simulink library "VentilatorLibrary"  (R2019b)
settings: Solver=VariableStepAuto  StartTime=0.0  StopTime=10.0  RelTol=1e-3
PreLoadFcn:
  | % Conversion factors
  | cmH2O_to_Pa = 98.0665;
  | L_to_m3 = 1e-3;
  | 
  | % Load thermodynamic data of N2, O2 and water vapor
  | load moistAirProperties
undefined symbols (not defined in the file): D_tube
libraries: fl_lib x109, simulink x2, HVAC_lib x1, nesl_utility x1
(part 2 of 2)

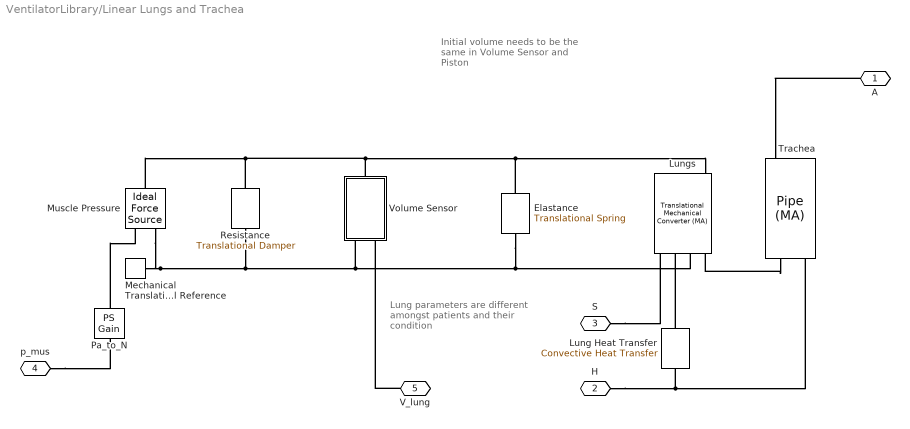
== system VentilatorLibrary/Linear Lungs and Trachea ==
  note: Lung parameters
      | are different
      | amongst patients
      | and their condition
  note: Initial volume needs
      | to be the same in
      | Volume Sensor
      | and Piston
  Elastance : fl_lib/Mechanical/Translational Elements/Translational Spring  spr_rate=E_respiratory*cmH2O_to_Pa/L_to_m3*A_interface^2 N/m  v_specify=off  v_priority=None  v=0 m/s  v_nominal_specify=off  v_nominal_unit=m/s  v_nominal_value=1  f_specify=off  f_priority=None  f=0 N  f_nominal_specify=off  f_nominal_unit=N  f_nominal_value=1  x_specify=on  x_priority=High  x=(vol_init - FRC)*L_to_m3/A_interface m  x_nominal_specify=off  x_nominal_unit=m  x_nominal_value=1
  Lung Heat Transfer : fl_lib/Thermal/Thermal Elements/Convective Heat Transfer  area=80 m^2  heat_tr_coeff=20 W/(m^2 * K)  T_specify=off  T_priority=None  T=0 K  T_nominal_specify=off  T_nominal_unit=K  T_nominal_value=1  Q_specify=off  Q_priority=None  Q=0 W  Q_nominal_specify=off  Q_nominal_unit=W  Q_nominal_value=1
  Lungs : fl_lib/Moist Air/Elements/Translational Mechanical Converter (MA)  mech_orientation=simscape.enum.posneg.positive  interface_area=A_interface m^2  length_init=vol_init* L_to_m3/A_interface m  dead_volume=1e-6 m^3  area_A=pi*D_trachea^2/4 m^2  pressure_spec=foundation.enum.pressure_spec.atmospheric  environment_pressure=0.101325 MPa  RH_ws=1  time_constant=1e-3 s  moisture_trace_gas_source=foundation.enum.moisture_trace_gas_source.controlled  moisture_source_spec=foundation.enum.moisture_source_spec.vapor  moisture_mass_flow=0 kg/s  moisture_temperature_spec=foundation.enum.temperature_spec.atmospheric  moisture_temperature=293.15 K  trace_gas_mass_flow=0 kg/s  trace_gas_temperature_spec=foundation.enum.temperature_spec.atmospheric  trace_gas_temperature=293.15 K  p_I_specify=on  p_I_priority=None  p_I=0.101325 MPa  p_I_nominal_specify=off  p_I_nominal_unit=MPa  p_I_nominal_value=1  T_I_specify=on  T_I_priority=High  T_I=T_init degC  T_I_nominal_specify=off  T_I_nominal_unit=K  T_I_nominal_value=1  RH_I_specify=on  RH_I_priority=High  RH_I=1  RH_I_nominal_specify=off  RH_I_nominal_unit=1  RH_I_nominal_value=1  x_w_I_specify=off  x_w_I_priority=None  x_w_I=0  x_w_I_nominal_specify=off  x_w_I_nominal_unit=1  x_w_I_nominal_value=1  y_w_I_specify=off  y_w_I_priority=None  y_w_I=0  y_w_I_nominal_specify=off  y_w_I_nominal_unit=1  y_w_I_nominal_value=1  HR_I_specify=off  HR_I_priority=None  HR_I=0  HR_I_nominal_specify=off  HR_I_nominal_unit=1  HR_I_nominal_value=1  x_g_I_specify=on  x_g_I_priority=None  x_g_I=0  x_g_I_nominal_specify=off  x_g_I_nominal_unit=1  x_g_I_nominal_value=1  y_g_I_specify=on  y_g_I_priority=High  y_g_I=0.7  y_g_I_nominal_specify=off  y_g_I_nominal_unit=1  y_g_I_nominal_value=1
      settings: SourceProductName=Simscape  SourceProductBaseCode=SS  InternalSimscapePortConfiguration="{\"Bottom\":[],\"Left\":[{\"id\":\"A\",\"label\":\"A\",\"type\":\"foundation.moist_air.moist_air\"},{\"id\":\"C\",\"label\":\"C\",\"type\":\"foundation.mechanical.translational.translational\"},{\"id\":\"H\",\"label\":\"H\",\"type\":\"foundation.thermal.thermal\"},{\"id\":\"S\",\"label\":\"S\",\"type\":\"foundation.moist_air.moist_air_source\"}],\"Right\":[{\"id\":\"R\",\"label\":\"R\",\"type\":\"foundation.mechanical.translational.translational\"},{\"id\":\"W\",\"label\":\"W\",\"type\":\"output\"},{\"id\":\"F\",\"label\":\"F\",\"type\":\"output\"}],\"Top\":[]}"
  Mechanical Translational Reference : fl_lib/Mechanical/Translational Elements/Mechanical Translational Reference
  Muscle Pressure : fl_lib/Mechanical/Mechanical Sources/Ideal Force Source
  Pa_to_N : fl_lib/Physical Signals/Functions/PS Gain  gain=A_interface N/Pa
  Resistance : fl_lib/Mechanical/Translational Elements/Translational Damper  D=(R_respiratory * cmH2O_to_Pa/ L_to_m3)*A_interface^2 N/(m/s)  v_specify=off  v_priority=None  v=0 m/s  v_nominal_specify=off  v_nominal_unit=m/s  v_nominal_value=1  f_specify=off  f_priority=None  f=0 N  f_nominal_specify=off  f_nominal_unit=N  f_nominal_value=1
  Trachea : fl_lib/Moist Air/Elements/Pipe (MA)  length=L_trachea m  area=pi*D_trachea^2/4 m^2  Dh=D_trachea m  length_add=0.1 m  roughness=15e-6 m  Re_lam=2000  Re_tur=4000  shape_factor=64  Nu_lam=3.66  RH_ws=1  time_constant=1e-3 s  moisture_trace_gas_source=foundation.enum.moisture_trace_gas_source.none  moisture_source_spec=foundation.enum.moisture_source_spec.vapor  moisture_mass_flow=0 kg/s  moisture_temperature_spec=foundation.enum.temperature_spec.atmospheric  moisture_temperature=293.15 K  trace_gas_mass_flow=0 kg/s  trace_gas_temperature_spec=foundation.enum.temperature_spec.atmospheric  trace_gas_temperature=293.15 K  p_I_specify=on  p_I_priority=None  p_I=0.101325 MPa  p_I_nominal_specify=off  p_I_nominal_unit=MPa  p_I_nominal_value=1  T_I_specify=on  T_I_priority=High  T_I=T_init degC  T_I_nominal_specify=off  T_I_nominal_unit=K  T_I_nominal_value=1  RH_I_specify=on  RH_I_priority=High  RH_I=1  RH_I_nominal_specify=off  RH_I_nominal_unit=1  RH_I_nominal_value=1  x_w_I_specify=off  x_w_I_priority=None  x_w_I=0  x_w_I_nominal_specify=off  x_w_I_nominal_unit=1  x_w_I_nominal_value=1  y_w_I_specify=off  y_w_I_priority=None  y_w_I=0  y_w_I_nominal_specify=off  y_w_I_nominal_unit=1  y_w_I_nominal_value=1  HR_I_specify=off  HR_I_priority=None  HR_I=0  HR_I_nominal_specify=off  HR_I_nominal_unit=1  HR_I_nominal_value=1  x_g_I_specify=on  x_g_I_priority=None  x_g_I=0  x_g_I_nominal_specify=off  x_g_I_nominal_unit=1  x_g_I_nominal_value=1  y_g_I_specify=on  y_g_I_priority=High  y_g_I=0.7  y_g_I_nominal_specify=off  y_g_I_nominal_unit=1  y_g_I_nominal_value=1
      settings: SourceProductName=Simscape  SourceProductBaseCode=SS
  Volume Sensor : Subsystem  mask(Volume Data){vol_init=vol_init}
      mask prompts: vol_init "Initial lung volume [L]"
      mask help: This subsystem reports the lung volume. Because the Interface cross-sectional area parameter in the lung model is set to 1 m^2, therefore 1 m of measured displacement is equivalent to 1 m^3 of lung volume and 1 N of measured force is equivalent to 1 Pa of pressure.
      mask init:
      | L_to_m3 = 1e-3;
  A : PMIOPort  Side=Right
  H : PMIOPort  Port=2  Side=Left
  S : PMIOPort  Port=3  Side=Left
  p_mus : PMIOPort  Port=4  Side=Left
  V_lung : PMIOPort  Port=5  Side=Right
  connections:
  Pa_to_N/RConn1 -- Muscle Pressure/RConn1
  p_mus/RConn1 -- Pa_to_N/LConn1
  V_lung/RConn1 -- Volume Sensor/RConn2
  S/RConn1 -- Lungs/LConn4
  A/RConn1 -- Trachea/RConn1
  Volume Sensor/RConn1 -- Resistance/RConn1 -- Muscle Pressure/RConn2 -- Mechanical Translational Reference/LConn1 -- Elastance/RConn1 -- Lungs/LConn2
  Lung Heat Transfer/LConn1 -- Lungs/LConn3
  Trachea/LConn2 -- Lung Heat Transfer/RConn1 -- H/RConn1
  Resistance/LConn1 -- Muscle Pressure/LConn1 -- Volume Sensor/LConn1 -- Elastance/LConn1 -- Lungs/RConn1
  Trachea/LConn1 -- Lungs/LConn1

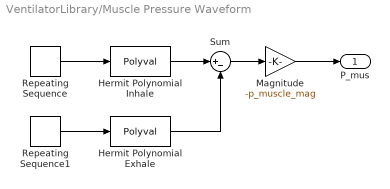
== system VentilatorLibrary/Muscle Pressure Waveform ==
  Hermit Polynomial Exhale : Polyval  Coefs=[-2, 3, 0, 0]
  Hermit Polynomial Inhale : Polyval  Coefs=[-2, 3, 0, 0]
  Magnitude : Gain  Gain=-p_muscle_mag
  Repeating Sequence : simulink/Sources/Repeating Sequence  rep_seq_t=[0, t_inhale, period]  rep_seq_y=[0, 1, 1]
  Repeating Sequence1 : simulink/Sources/Repeating Sequence  rep_seq_t=[0, t_inhale, t_inhale+t_exhale, period]  rep_seq_y=[0, 0, 1, 1]
  Sum : Sum  Inputs=|+-
  P_mus : Outport  VectorParamsAs1DForOutWhenUnconnected=off
  wires:
  Magnitude/1 -> P_mus/1
  Hermit Polynomial Inhale/1 -> Sum/1
  Repeating Sequence/1 -> Hermit Polynomial Inhale/1
  Repeating Sequence1/1 -> Hermit Polynomial Exhale/1
  Sum/1 -> Magnitude/1
  Hermit Polynomial Exhale/1 -> Sum/2

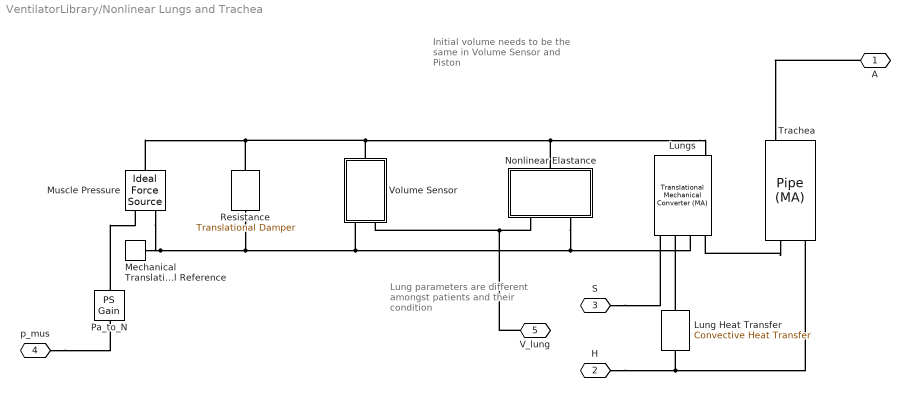
== system VentilatorLibrary/Nonlinear Lungs and Trachea ==
  note: Initial volume needs
      | to be the same in
      | Volume Sensor
      | and Piston
  note: Lung parameters
      | are different
      | amongst patients
      | and their condition
  Lung Heat Transfer : fl_lib/Thermal/Thermal Elements/Convective Heat Transfer  area=80 m^2  heat_tr_coeff=20 W/(m^2 * K)  T_specify=off  T_priority=None  T=0 K  T_nominal_specify=off  T_nominal_unit=K  T_nominal_value=1  Q_specify=off  Q_priority=None  Q=0 W  Q_nominal_specify=off  Q_nominal_unit=W  Q_nominal_value=1
  Lungs : fl_lib/Moist Air/Elements/Translational Mechanical Converter (MA)  mech_orientation=simscape.enum.posneg.positive  interface_area=A_interface m^2  length_init=vol_init* L_to_m3/A_interface m  dead_volume=1e-6 m^3  area_A=pi*D_trachea^2/4 m^2  pressure_spec=foundation.enum.pressure_spec.atmospheric  environment_pressure=0.101325 MPa  RH_ws=1  time_constant=1e-3 s  moisture_trace_gas_source=foundation.enum.moisture_trace_gas_source.controlled  moisture_source_spec=foundation.enum.moisture_source_spec.vapor  moisture_mass_flow=0 kg/s  moisture_temperature_spec=foundation.enum.temperature_spec.atmospheric  moisture_temperature=293.15 K  trace_gas_mass_flow=0 kg/s  trace_gas_temperature_spec=foundation.enum.temperature_spec.atmospheric  trace_gas_temperature=293.15 K  p_I_specify=on  p_I_priority=None  p_I=0.101325 MPa  p_I_nominal_specify=off  p_I_nominal_unit=MPa  p_I_nominal_value=1  T_I_specify=on  T_I_priority=High  T_I=T_init degC  T_I_nominal_specify=off  T_I_nominal_unit=K  T_I_nominal_value=1  RH_I_specify=on  RH_I_priority=High  RH_I=1  RH_I_nominal_specify=off  RH_I_nominal_unit=1  RH_I_nominal_value=1  x_w_I_specify=off  x_w_I_priority=None  x_w_I=0  x_w_I_nominal_specify=off  x_w_I_nominal_unit=1  x_w_I_nominal_value=1  y_w_I_specify=off  y_w_I_priority=None  y_w_I=0  y_w_I_nominal_specify=off  y_w_I_nominal_unit=1  y_w_I_nominal_value=1  HR_I_specify=off  HR_I_priority=None  HR_I=0  HR_I_nominal_specify=off  HR_I_nominal_unit=1  HR_I_nominal_value=1  x_g_I_specify=on  x_g_I_priority=None  x_g_I=0  x_g_I_nominal_specify=off  x_g_I_nominal_unit=1  x_g_I_nominal_value=1  y_g_I_specify=on  y_g_I_priority=High  y_g_I=0.7  y_g_I_nominal_specify=off  y_g_I_nominal_unit=1  y_g_I_nominal_value=1
      settings: SourceProductName=Simscape  SourceProductBaseCode=SS  InternalSimscapePortConfiguration="{\"Bottom\":[],\"Left\":[{\"id\":\"A\",\"label\":\"A\",\"type\":\"foundation.moist_air.moist_air\"},{\"id\":\"C\",\"label\":\"C\",\"type\":\"foundation.mechanical.translational.translational\"},{\"id\":\"H\",\"label\":\"H\",\"type\":\"foundation.thermal.thermal\"},{\"id\":\"S\",\"label\":\"S\",\"type\":\"foundation.moist_air.moist_air_source\"}],\"Right\":[{\"id\":\"R\",\"label\":\"R\",\"type\":\"foundation.mechanical.translational.translational\"},{\"id\":\"W\",\"label\":\"W\",\"type\":\"output\"},{\"id\":\"F\",\"label\":\"F\",\"type\":\"output\"}],\"Top\":[]}"
  Mechanical Translational Reference : fl_lib/Mechanical/Translational Elements/Mechanical Translational Reference
  Muscle Pressure : fl_lib/Mechanical/Mechanical Sources/Ideal Force Source
  Nonlinear Elastance : Subsystem  mask{Vmax=Vmax, E_respiratory=E_respiratory, FRC=FRC}
      mask prompts: Vmax "Lung capacity [L]:"; E_respiratory "Elastance at equilibrium volume [cmH2O/L]"; FRC "Functional Residual Capacity (equilibrium volume) [L]:"
      mask Display: disp('F=k2*tan(k1*x)')
  Pa_to_N : fl_lib/Physical Signals/Functions/PS Gain  gain=A_interface N/Pa
  Resistance : fl_lib/Mechanical/Translational Elements/Translational Damper  D=(R_respiratory * cmH2O_to_Pa/ L_to_m3)*A_interface^2 N/(m/s)  v_specify=off  v_priority=None  v=0 m/s  v_nominal_specify=off  v_nominal_unit=m/s  v_nominal_value=1  f_specify=off  f_priority=None  f=0 N  f_nominal_specify=off  f_nominal_unit=N  f_nominal_value=1
  Trachea : fl_lib/Moist Air/Elements/Pipe (MA)  length=L_trachea m  area=pi*D_trachea^2/4 m^2  Dh=D_trachea m  length_add=0.1 m  roughness=15e-6 m  Re_lam=2000  Re_tur=4000  shape_factor=64  Nu_lam=3.66  RH_ws=1  time_constant=1e-3 s  moisture_trace_gas_source=foundation.enum.moisture_trace_gas_source.none  moisture_source_spec=foundation.enum.moisture_source_spec.vapor  moisture_mass_flow=0 kg/s  moisture_temperature_spec=foundation.enum.temperature_spec.atmospheric  moisture_temperature=293.15 K  trace_gas_mass_flow=0 kg/s  trace_gas_temperature_spec=foundation.enum.temperature_spec.atmospheric  trace_gas_temperature=293.15 K  p_I_specify=on  p_I_priority=None  p_I=0.101325 MPa  p_I_nominal_specify=off  p_I_nominal_unit=MPa  p_I_nominal_value=1  T_I_specify=on  T_I_priority=High  T_I=T_init degC  T_I_nominal_specify=off  T_I_nominal_unit=K  T_I_nominal_value=1  RH_I_specify=on  RH_I_priority=High  RH_I=1  RH_I_nominal_specify=off  RH_I_nominal_unit=1  RH_I_nominal_value=1  x_w_I_specify=off  x_w_I_priority=None  x_w_I=0  x_w_I_nominal_specify=off  x_w_I_nominal_unit=1  x_w_I_nominal_value=1  y_w_I_specify=off  y_w_I_priority=None  y_w_I=0  y_w_I_nominal_specify=off  y_w_I_nominal_unit=1  y_w_I_nominal_value=1  HR_I_specify=off  HR_I_priority=None  HR_I=0  HR_I_nominal_specify=off  HR_I_nominal_unit=1  HR_I_nominal_value=1  x_g_I_specify=on  x_g_I_priority=None  x_g_I=0  x_g_I_nominal_specify=off  x_g_I_nominal_unit=1  x_g_I_nominal_value=1  y_g_I_specify=on  y_g_I_priority=High  y_g_I=0.7  y_g_I_nominal_specify=off  y_g_I_nominal_unit=1  y_g_I_nominal_value=1
      settings: SourceProductName=Simscape  SourceProductBaseCode=SS
  Volume Sensor : Subsystem  mask(Volume Data){vol_init=vol_init}
      mask prompts: vol_init "Initial lung volume [L]"
      mask help: This subsystem reports the lung volume. Because the Interface cross-sectional area parameter in the lung model is set to 1 m^2, therefore 1 m of measured displacement is equivalent to 1 m^3 of lung volume and 1 N of measured force is equivalent to 1 Pa of pressure.
      mask init:
      | L_to_m3 = 1e-3
  A : PMIOPort  Side=Right
  H : PMIOPort  Port=2  Side=Left
  S : PMIOPort  Port=3  Side=Left
  p_mus : PMIOPort  Port=4  Side=Left
  V_lung : PMIOPort  Port=5  Side=Right
  connections:
  Trachea/LConn1 -- Lungs/LConn1
  Lungs/RConn1 -- Volume Sensor/LConn1 -- Muscle Pressure/LConn1 -- Resistance/LConn1 -- Nonlinear Elastance/LConn1
  H/RConn1 -- Lung Heat Transfer/RConn1 -- Trachea/LConn2
  Lung Heat Transfer/LConn1 -- Lungs/LConn3
  Lungs/LConn2 -- Mechanical Translational Reference/LConn1 -- Muscle Pressure/RConn2 -- Resistance/RConn1 -- Volume Sensor/RConn1 -- Nonlinear Elastance/RConn2
  A/RConn1 -- Trachea/RConn1
  S/RConn1 -- Lungs/LConn4
  Nonlinear Elastance/RConn1 -- Volume Sensor/RConn2 -- V_lung/RConn1
  p_mus/RConn1 -- Pa_to_N/LConn1
  Pa_to_N/RConn1 -- Muscle Pressure/RConn1

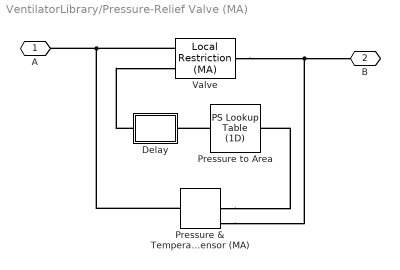
== system VentilatorLibrary/Pressure-Relief Valve (MA) ==
  Delay : Subsystem  mask{tau=tau, x0=A_leak}
      mask prompts: tau "Time constant (s)"; x0 "Initial output"
  Pressure & Temperature Sensor (MA) : fl_lib/Moist Air/Sensors/Pressure & Temperature Sensor (MA)
      settings: SourceProductName=Simscape  SourceProductBaseCode=SS  InternalSimscapePortConfiguration="{\"Bottom\":[],\"Left\":[{\"id\":\"A\",\"label\":\"A\",\"type\":\"foundation.moist_air.moist_air\"}],\"Right\":[{\"id\":\"B\",\"label\":\"B\",\"type\":\"foundation.moist_air.moist_air\"},{\"id\":\"P\",\"label\":\"P\",\"type\":\"output\"},{\"id\":\"T\",\"label\":\"T\",\"type\":\"output\"}],\"Top\":[]}"
  Pressure to Area : fl_lib/Physical Signals/Lookup Tables/PS Lookup Table (1D)  x=[0 p_set p_max p_max+1] Pa  f=[A_leak, A_leak, A_max, A_max] m^2  interp_method=simscape.enum.interpolation.linear  extrap_method=simscape.enum.extrapolation.nearest
      settings: SourceProductName=Simscape  SourceProductBaseCode=SS
  Valve : fl_lib/Moist Air/Elements/Local Restriction (MA)  restriction_type=foundation.enum.restriction_type.variable  restriction_area=0.001 m^2  min_area=A_leak/2 m^2  max_area=(A_max + A_port)/2 m^2  area=A_port m^2  Cd=Cd  B_lam=0.999
      settings: SourceProductName=Simscape  SourceProductBaseCode=SS
  A : PMIOPort  Side=Left
  B : PMIOPort  Port=2  Side=Right
  connections:
  Pressure & Temperature Sensor (MA)/LConn1 -- Valve/LConn1 -- A/RConn1
  Pressure & Temperature Sensor (MA)/RConn1 -- Valve/RConn1 -- B/RConn1
  Pressure & Temperature Sensor (MA)/RConn2 -- Pressure to Area/LConn1
  Pressure to Area/RConn1 -- Delay/LConn1
  Delay/RConn1 -- Valve/LConn2

== system VentilatorLibrary/Proportional Valve (MA) ==
  Local Restriction (MA) : fl_lib/Moist Air/Elements/Local Restriction (MA)  restriction_type=foundation.enum.restriction_type.variable  restriction_area=0.001 m^2  min_area=area_leak in^2  max_area=area_max in^2  area=area_A in^2  Cd=Cd  B_lam=pr
      settings: SourceProductName=Simscape  SourceProductBaseCode=SS
  Map Voltage to Area : fl_lib/Physical Signals/Functions/PS Gain  gain=area_max/Vmax in^2/V
  Valve Dynamics : Subsystem  mask{tau=tau, x0=area_leak}
      mask prompts: tau "Time constant (s)"; x0 "Initial output [in^2]"
  Vref : PMIOPort  Side=Left
  B : PMIOPort  Port=2  Side=Right
  A : PMIOPort  Port=3  Side=Left
  connections:
  Local Restriction (MA)/RConn1 -- B/RConn1
  A/RConn1 -- Local Restriction (MA)/LConn1
  Vref/RConn1 -- Map Voltage to Area/LConn1
  Valve Dynamics/RConn1 -- Local Restriction (MA)/LConn2
  Map Voltage to Area/RConn1 -- Valve Dynamics/LConn1

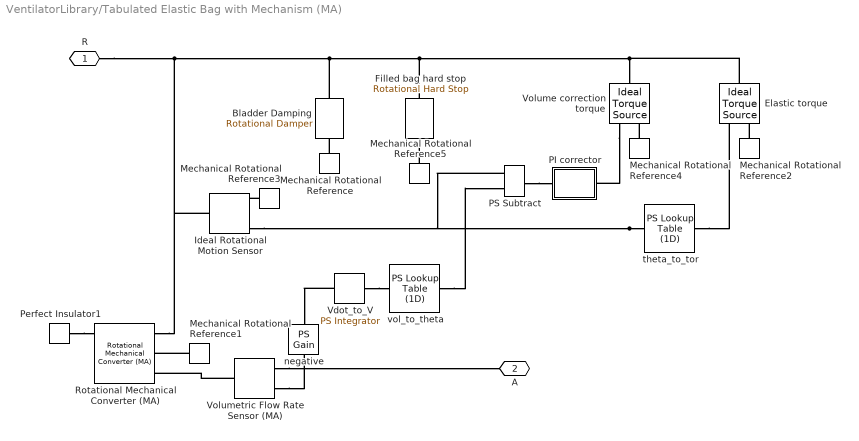
== system VentilatorLibrary/Tabulated Elastic Bag with Mechanism (MA) ==
  Bladder Damping : fl_lib/Mechanical/Rotational Elements/Rotational Damper  D=damp N*m/(rad/s)  w_specify=off  w_priority=None  w=0 rad/s  w_nominal_specify=off  w_nominal_unit=rad/s  w_nominal_value=1  t_specify=off  t_priority=None  t=0 N*m  t_nominal_specify=off  t_nominal_unit=N*m  t_nominal_value=1
  Elastic torque : fl_lib/Mechanical/Mechanical Sources/Ideal Torque Source
  Filled bag hard stop : fl_lib/Mechanical/Rotational Elements/Rotational Hard Stop  upper_bnd=max(theta_TLU) rad  lower_bnd=min(theta_TLU) rad  stiff_up=Kfull N*m/rad  stiff_low=Kfull N*m/rad  D_up=0.01 N*m/(rad/s)  D_low=0.01 N*m/(rad/s)  model=simscape.enum.hardstop.smooth  transition=(max(theta_TLU) - min(theta_TLU))/10 rad  w_specify=off  w_priority=None  w=0 rad/s  w_nominal_specify=off  w_nominal_unit=rad/s  w_nominal_value=1  t_specify=off  t_priority=None  t=0 N*m  t_nominal_specify=off  t_nominal_unit=N*m  t_nominal_value=1  phi_specify=on  phi_priority=High  phi=theta_init rad  phi_nominal_specify=off  phi_nominal_unit=rad  phi_nominal_value=1
      settings: SourceProductName=Simscape  SourceProductBaseCode=SS
  Ideal Rotational Motion Sensor : fl_lib/Mechanical/Mechanical Sensors/Ideal Rotational Motion Sensor  offset=theta_init rad
  Mechanical Rotational Reference{,1..5} (6 alike) : fl_lib/Mechanical/Rotational Elements/Mechanical Rotational Reference
  PI corrector : Subsystem  mask{tau=tau, K=Kcorr}
      mask prompts: tau "Time constant (s)"; K "Proportional gain [N*m/rad]"
  PS Subtract : fl_lib/Physical Signals/Functions/PS Subtract
      settings: SourceProductName=Simscape
  Perfect Insulator1 : fl_lib/Thermal/Thermal Elements/Perfect Insulator  T_specify=off  T_priority=None  T=0 K  T_nominal_specify=off  T_nominal_unit=K  T_nominal_value=1
      settings: SourceProductName=Simscape
  Rotational Mechanical Converter (MA) : fl_lib/Moist Air/Elements/Rotational Mechanical Converter (MA)  mech_orientation=simscape.enum.posneg.positive  volume_displacement=(max(V_TLU)-min(V_TLU))/(max(theta_TLU)-min(theta_TLU)) l/rad  theta_init=theta_init rad  dead_volume=min(V_TLU) l  area_A=area_A m^2  pressure_spec=foundation.enum.pressure_spec.atmospheric  environment_pressure=0.101325 MPa  RH_ws=1  time_constant=1e-3 s  moisture_trace_gas_source=foundation.enum.moisture_trace_gas_source.none  moisture_source_spec=foundation.enum.moisture_source_spec.vapor  moisture_mass_flow=0 kg/s  moisture_temperature_spec=foundation.enum.temperature_spec.atmospheric  moisture_temperature=293.15 K  trace_gas_mass_flow=0 kg/s  trace_gas_temperature_spec=foundation.enum.temperature_spec.atmospheric  trace_gas_temperature=293.15 K  p_I_specify=on  p_I_priority=High  p_I=p_init bar  p_I_nominal_specify=off  p_I_nominal_unit=MPa  p_I_nominal_value=1  T_I_specify=on  T_I_priority=High  T_I=T_init K  T_I_nominal_specify=off  T_I_nominal_unit=K  T_I_nominal_value=1  RH_I_specify=on  RH_I_priority=High  RH_I=hum_init  RH_I_nominal_specify=off  RH_I_nominal_unit=1  RH_I_nominal_value=1  x_w_I_specify=off  x_w_I_priority=None  x_w_I=0  x_w_I_nominal_specify=off  x_w_I_nominal_unit=1  x_w_I_nominal_value=1  y_w_I_specify=off  y_w_I_priority=None  y_w_I=0  y_w_I_nominal_specify=off  y_w_I_nominal_unit=1  y_w_I_nominal_value=1  HR_I_specify=off  HR_I_priority=None  HR_I=0  HR_I_nominal_specify=off  HR_I_nominal_unit=1  HR_I_nominal_value=1  x_g_I_specify=on  x_g_I_priority=None  x_g_I=0  x_g_I_nominal_specify=off  x_g_I_nominal_unit=1  x_g_I_nominal_value=1  y_g_I_specify=on  y_g_I_priority=High  y_g_I=y_tg_init  y_g_I_nominal_specify=off  y_g_I_nominal_unit=1  y_g_I_nominal_value=1
      settings: SourceProductName=Simscape  SourceProductBaseCode=SS  InternalSimscapePortConfiguration="{\"Bottom\":[],\"Left\":[{\"id\":\"A\",\"label\":\"A\",\"type\":\"foundation.moist_air.moist_air\"},{\"id\":\"C\",\"label\":\"C\",\"type\":\"foundation.mechanical.rotational.rotational\"},{\"id\":\"R\",\"label\":\"R\",\"type\":\"foundation.mechanical.rotational.rotational\"}],\"Right\":[{\"id\":\"W\",\"label\":\"W\",\"type\":\"output\"},{\"id\":\"F\",\"label\":\"F\",\"type\":\"output\"},{\"id\":\"H\",\"label\":\"H\",\"type\":\"foundation.thermal.thermal\"}],\"Top\":[]}"
  Vdot_to_V : fl_lib/Physical Signals/Linear Operators/PS Integrator  x0=interp1(theta_TLU, V_TLU, theta_init) l
      settings: SourceProductName=Simscape  SourceProductBaseCode=SS
  Volume correction torque : fl_lib/Mechanical/Mechanical Sources/Ideal Torque Source
  Volumetric Flow Rate Sensor (MA) : fl_lib/Moist Air/Sensors/Volumetric Flow Rate Sensor (MA)  volumetric_flow_conditions=foundation.enum.volumetric_flow_conditions.actual  p_std=0.101325 MPa  T_std=20 degC  RH_std=0.65
      settings: SourceProductName=Simscape  SourceProductBaseCode=SS  InternalSimscapePortConfiguration="{\"Bottom\":[],\"Left\":[{\"id\":\"A\",\"label\":\"A\",\"type\":\"foundation.moist_air.moist_air\"}],\"Right\":[{\"id\":\"B\",\"label\":\"B\",\"type\":\"foundation.moist_air.moist_air\"},{\"id\":\"V\",\"label\":\"V\",\"type\":\"output\"}],\"Top\":[]}"
  negative : fl_lib/Physical Signals/Functions/PS Gain  gain=-1
  theta_to_tor : fl_lib/Physical Signals/Lookup Tables/PS Lookup Table (1D)  x=theta_TLU rad  f=tor_TLU N*m  interp_method=simscape.enum.interpolation.smooth  extrap_method=simscape.enum.extrapolation.linear
      settings: SourceProductName=Simscape  SourceProductBaseCode=SS
  vol_to_theta : fl_lib/Physical Signals/Lookup Tables/PS Lookup Table (1D)  x=V_TLU l  f=theta_TLU rad  interp_method=simscape.enum.interpolation.smooth  extrap_method=simscape.enum.extrapolation.linear
      settings: SourceProductName=Simscape  SourceProductBaseCode=SS
  R : PMIOPort  Side=Left
  A : PMIOPort  Port=2  Side=Right
  connections:
  Perfect Insulator1/LConn1 -- Rotational Mechanical Converter (MA)/RConn3
  theta_to_tor/RConn1 -- Elastic torque/RConn1
  Elastic torque/LConn1 -- Volume correction torque/LConn1 -- Filled bag hard stop/LConn1 -- Bladder Damping/LConn1 -- Rotational Mechanical Converter (MA)/LConn3 -- Ideal Rotational Motion Sensor/LConn1 -- R/RConn1
  Mechanical Rotational Reference1/LConn1 -- Rotational Mechanical Converter (MA)/LConn2
  Mechanical Rotational Reference2/LConn1 -- Elastic torque/RConn2
  Volumetric Flow Rate Sensor (MA)/RConn2 -- negative/LConn1
  Vdot_to_V/RConn1 -- vol_to_theta/LConn1
  Mechanical Rotational Reference3/LConn1 -- Ideal Rotational Motion Sensor/RConn1
  Mechanical Rotational Reference4/LConn1 -- Volume correction torque/RConn2
  Volume correction torque/RConn1 -- PI corrector/RConn1
  theta_to_tor/LConn1 -- Ideal Rotational Motion Sensor/RConn3 -- PS Subtract/LConn2
  Volumetric Flow Rate Sensor (MA)/LConn1 -- Rotational Mechanical Converter (MA)/LConn1
  Volumetric Flow Rate Sensor (MA)/RConn1 -- A/RConn1
  Vdot_to_V/LConn1 -- negative/RConn1
  PS Subtract/RConn1 -- PI corrector/LConn1
  vol_to_theta/RConn1 -- PS Subtract/LConn1
  Mechanical Rotational Reference/LConn1 -- Bladder Damping/RConn1
  Mechanical Rotational Reference5/LConn1 -- Filled bag hard stop/RConn1

== system VentilatorLibrary/Tabulated Volumetric Flow Source (MA) ==
  PS Lookup Table (1D) : fl_lib/Physical Signals/Lookup Tables/PS Lookup Table (1D)  x="p_diff_TLU*1e-3  bar"  f=V_TLU m^3/hr  interp_method=simscape.enum.interpolation.linear  extrap_method=simscape.enum.extrapolation.linear
      settings: SourceProductName=Simscape  SourceProductBaseCode=SS
  PS Saturation : fl_lib/Physical Signals/Nonlinear Operators/PS Saturation  upper_limit=inf m^3/hr  lower_limit=0 m^3/hr
      settings: SourceProductName=Simscape  SourceProductBaseCode=SS
  Pressure & Temperature Sensor (MA) : fl_lib/Moist Air/Sensors/Pressure & Temperature Sensor (MA)
      settings: SourceProductName=Simscape  SourceProductBaseCode=SS  InternalSimscapePortConfiguration="{\"Bottom\":[],\"Left\":[{\"id\":\"A\",\"label\":\"A\",\"type\":\"foundation.moist_air.moist_air\"}],\"Right\":[{\"id\":\"B\",\"label\":\"B\",\"type\":\"foundation.moist_air.moist_air\"},{\"id\":\"P\",\"label\":\"P\",\"type\":\"output\"},{\"id\":\"T\",\"label\":\"T\",\"type\":\"output\"}],\"Top\":[]}"
  Volumetric Supply : fl_lib/Moist Air/Sources/Controlled Volumetric Flow Rate Source (MA)  power_spec=foundation.enum.power_spec.isentropic  volumetric_flow_conditions=foundation.enum.volumetric_flow_conditions.actual  p_std=0.101325 MPa  T_std=20 degC  RH_std=0.65  area_A=area_A m^2  area_B=area_B m^2
      settings: SourceProductName=Simscape  SourceProductBaseCode=SS  InternalSimscapePortConfiguration="{\"Bottom\":[],\"Left\":[{\"id\":\"A\",\"label\":\"A\",\"type\":\"foundation.moist_air.moist_air\"},{\"id\":\"V\",\"label\":\"V\",\"type\":\"input\"}],\"Right\":[{\"id\":\"B\",\"label\":\"B\",\"type\":\"foundation.moist_air.moist_air\"}],\"Top\":[]}"
  A : PMIOPort  Side=Left
  B : PMIOPort  Port=2  Side=Right
  connections:
  PS Saturation/RConn1 -- Volumetric Supply/LConn2
  Pressure & Temperature Sensor (MA)/RConn2 -- PS Lookup Table (1D)/LConn1
  Pressure & Temperature Sensor (MA)/RConn1 -- A/RConn1 -- Volumetric Supply/LConn1
  Volumetric Supply/RConn1 -- B/RConn1 -- Pressure & Temperature Sensor (MA)/LConn1
  PS Saturation/LConn1 -- PS Lookup Table (1D)/RConn1

== system VentilatorLibrary/Check Valve (MA)/Delay ==
  PS Gain : fl_lib/Physical Signals/Functions/PS Gain  gain=1/tau 1/s
  PS Integrator : fl_lib/Physical Signals/Linear Operators/PS Integrator  x0=x0 m^2
      settings: SourceProductName=Simscape  SourceProductBaseCode=SS
  PS Subtract : fl_lib/Physical Signals/Functions/PS Subtract
      settings: SourceProductName=Simscape
  A : PMIOPort  Side=Left
  B : PMIOPort  Port=2  Side=Right
  connections:
  PS Integrator/RConn1 -- PS Subtract/LConn2 -- B/RConn1
  PS Subtract/RConn1 -- PS Gain/LConn1
  PS Subtract/LConn1 -- A/RConn1
  PS Integrator/LConn1 -- PS Gain/RConn1

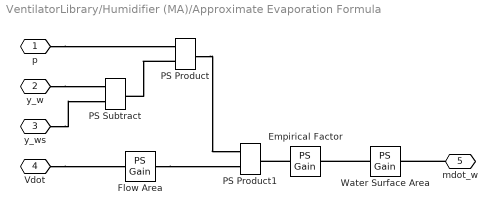
== system VentilatorLibrary/Humidifier (MA)/Approximate Evaporation Formula ==
  Empirical Factor : fl_lib/Physical Signals/Functions/PS Gain  gain=5e-8 kg/J
  Flow Area : fl_lib/Physical Signals/Functions/PS Gain  gain=1 / (pi*D_tube^2/4) 1/m^2
  PS Product : fl_lib/Physical Signals/Functions/PS Product
      settings: SourceProductName=Simscape
  PS Product1 : fl_lib/Physical Signals/Functions/PS Product
      settings: SourceProductName=Simscape
  PS Subtract : fl_lib/Physical Signals/Functions/PS Subtract
      settings: SourceProductName=Simscape
  Water Surface Area : fl_lib/Physical Signals/Functions/PS Gain  gain=A_humidifier m^2
  p : PMIOPort  Side=Left
  y_w : PMIOPort  Port=2  Side=Left
  y_ws : PMIOPort  Port=3  Side=Left
  Vdot : PMIOPort  Port=4  Side=Left
  mdot_w : PMIOPort  Port=5  Side=Right
  connections:
  y_w/RConn1 -- PS Subtract/LConn2
  y_ws/RConn1 -- PS Subtract/LConn1
  p/RConn1 -- PS Product/LConn1
  PS Product/LConn2 -- PS Subtract/RConn1
  PS Product/RConn1 -- PS Product1/LConn1
  Flow Area/RConn1 -- PS Product1/LConn2
  Empirical Factor/LConn1 -- PS Product1/RConn1
  Water Surface Area/LConn1 -- Empirical Factor/RConn1
  mdot_w/RConn1 -- Water Surface Area/RConn1
  Vdot/RConn1 -- Flow Area/LConn1

== system VentilatorLibrary/Linear Lungs and Trachea/Volume Sensor ==
  Ideal Translational Motion Sensor : fl_lib/Mechanical/Mechanical Sensors/Ideal Translational Motion Sensor  offset=vol_init*L_to_m3/A_interface m
  pos_to_vol : fl_lib/Physical Signals/Functions/PS Gain  gain=A_interface m^2
  R : PMIOPort  Side=Left
  C : PMIOPort  Port=2  Side=Right
  V_lung : PMIOPort  Port=3  Side=Right
  connections:
  V_lung/RConn1 -- pos_to_vol/RConn1
  Ideal Translational Motion Sensor/RConn3 -- pos_to_vol/LConn1
  Ideal Translational Motion Sensor/RConn1 -- C/RConn1
  Ideal Translational Motion Sensor/LConn1 -- R/RConn1

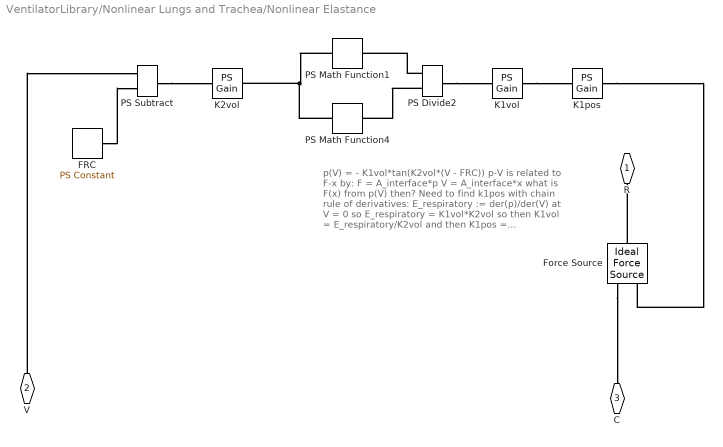
== system VentilatorLibrary/Nonlinear Lungs and Trachea/Nonlinear Elastance ==
  note: p(V) = - K1vol*tan(K2vol*(V - FRC))
      |
      | p-V is related to F-x by:
      |
      | F = A_interface*p
      | V = A_interface*x
      |
      | what is F(x) from p(V) then?
      |
      | Need to find k1pos with chain rule of derivatives:
      |
      | E_respiratory := der(p)/der(V) at V = 0
      | so E_respiratory = K1vol*K2vol
      | so then K1vol = E_respiratory/K2vol
      | and then K1pos = K1vol*A_interface,
      | because F = A_interface*p
  FRC : fl_lib/Physical Signals/Sources/PS Constant  constant=FRC l
  Force Source : fl_lib/Mechanical/Mechanical Sources/Ideal Force Source
      settings: SourceProductBaseCode=MT,SS
  K1pos : fl_lib/Physical Signals/Functions/PS Gain  gain=A_interface m^2
  K1vol : fl_lib/Physical Signals/Functions/PS Gain  gain=-(E_respiratory*cmH2O_to_Pa*(Vmax-FRC))/(pi/2) Pa
  K2vol : fl_lib/Physical Signals/Functions/PS Gain  gain=(pi/2)/(Vmax-FRC) rad/l
  PS Divide2 : fl_lib/Physical Signals/Functions/PS Divide
      settings: SourceProductBaseCode=SS
  PS Math Function1 : fl_lib/Physical Signals/Functions/PS Math Function  fcn_choice=foundation.enum.math_function.sin
      settings: SourceProductBaseCode=SS
  PS Math Function4 : fl_lib/Physical Signals/Functions/PS Math Function  fcn_choice=foundation.enum.math_function.cos
      settings: SourceProductBaseCode=SS
  PS Subtract : fl_lib/Physical Signals/Functions/PS Subtract
      settings: SourceProductName=Simscape
  R : PMIOPort  Side=Left
  V : PMIOPort  Port=2  Side=Right
  C : PMIOPort  Port=3  Side=Right
  connections:
  Force Source/LConn1 -- R/RConn1
  Force Source/RConn2 -- C/RConn1
  PS Math Function4/LConn1 -- PS Math Function1/LConn1 -- K2vol/RConn1
  PS Divide2/LConn1 -- PS Math Function1/RConn1
  PS Divide2/LConn2 -- PS Math Function4/RConn1
  PS Divide2/RConn1 -- K1vol/LConn1
  FRC/RConn1 -- PS Subtract/LConn2
  V/RConn1 -- PS Subtract/LConn1
  PS Subtract/RConn1 -- K2vol/LConn1
  K1vol/RConn1 -- K1pos/LConn1
  K1pos/RConn1 -- Force Source/RConn1

== system VentilatorLibrary/Nonlinear Lungs and Trachea/Volume Sensor ==
  Ideal Translational Motion Sensor : fl_lib/Mechanical/Mechanical Sensors/Ideal Translational Motion Sensor  offset=vol_init*L_to_m3/A_interface m
  pos_to_vol : fl_lib/Physical Signals/Functions/PS Gain  gain=A_interface m^2
  R : PMIOPort  Side=Left
  C : PMIOPort  Port=2  Side=Right
  V_lung : PMIOPort  Port=3  Side=Right
  connections:
  Ideal Translational Motion Sensor/LConn1 -- R/RConn1
  Ideal Translational Motion Sensor/RConn1 -- C/RConn1
  Ideal Translational Motion Sensor/RConn3 -- pos_to_vol/LConn1
  V_lung/RConn1 -- pos_to_vol/RConn1

== system VentilatorLibrary/Pressure-Relief Valve (MA)/Delay ==
  PS Gain : fl_lib/Physical Signals/Functions/PS Gain  gain=1/tau 1/s
  PS Integrator : fl_lib/Physical Signals/Linear Operators/PS Integrator  x0=x0 m^2
      settings: SourceProductName=Simscape  SourceProductBaseCode=SS
  PS Subtract : fl_lib/Physical Signals/Functions/PS Subtract
      settings: SourceProductName=Simscape
  A : PMIOPort  Side=Left
  B : PMIOPort  Port=2  Side=Right
  connections:
  PS Integrator/RConn1 -- PS Subtract/LConn2 -- B/RConn1
  PS Subtract/RConn1 -- PS Gain/LConn1
  PS Subtract/LConn1 -- A/RConn1
  PS Integrator/LConn1 -- PS Gain/RConn1

== system VentilatorLibrary/Proportional Valve (MA)/Valve Dynamics ==
  PS Gain : fl_lib/Physical Signals/Functions/PS Gain  gain=1/tau 1/s
  PS Integrator : fl_lib/Physical Signals/Linear Operators/PS Integrator  x0=x0 in^2
      settings: SourceProductName=Simscape  SourceProductBaseCode=SS
  PS Subtract : fl_lib/Physical Signals/Functions/PS Subtract
      settings: SourceProductName=Simscape
  A : PMIOPort  Side=Left
  B : PMIOPort  Port=2  Side=Right
  connections:
  PS Integrator/RConn1 -- PS Subtract/LConn2 -- B/RConn1
  PS Subtract/RConn1 -- PS Gain/LConn1
  PS Subtract/LConn1 -- A/RConn1
  PS Integrator/LConn1 -- PS Gain/RConn1

== system VentilatorLibrary/Tabulated Elastic Bag with Mechanism (MA)/PI corrector ==
  Kcorr : fl_lib/Physical Signals/Functions/PS Gain  gain=Kcorr N*m/rad
  PS Gain : fl_lib/Physical Signals/Functions/PS Gain  gain=1/tau 1/s
  PS Integrator : fl_lib/Physical Signals/Linear Operators/PS Integrator  x0=0 deg
      settings: SourceProductName=Simscape  SourceProductBaseCode=SS
  PS Subtract : fl_lib/Physical Signals/Functions/PS Subtract
      settings: SourceProductName=Simscape
  err : PMIOPort  Side=Left
  tor : PMIOPort  Port=2  Side=Right
  connections:
  Kcorr/RConn1 -- tor/RConn1
  PS Subtract/RConn1 -- PS Gain/LConn1
  PS Subtract/LConn1 -- err/RConn1
  PS Integrator/LConn1 -- PS Gain/RConn1
  PS Integrator/RConn1 -- Kcorr/LConn1 -- PS Subtract/LConn2
